simulink model "prova"  (R2023b)
settings: Solver=ode4  StartTime=0.0  StopTime=tf  FixedStep=t_step  RelTol=1e-3
values from neighbouring files (symbols this model uses):
  ARW = ARW*[1 1 1]'    [gyroscope.m]
  bias = bias*[1 1 1]'    [gyroscope.m]
  I = [Ix 0 0; 0 Iy 0; 0 0 Iz]    [gyroscope.m]
  I_inv = inv(I)    [gyroscope.m]
undefined symbols (not defined in the file or in its folder): A_1, A_2, A_3, A_4, A_5, A_6, alpha, DCM_eci_per, e, FS, H0, h_r_0, i, I_RW, I_vector_RW, inc_tot, InitialTrueAnomalyOfEarth, j_b, matrix_RW_config, matrix_RW_config_inv, mu_E, N_1, N_2, N_3, N_4, N_5, N_6, n_e, p, q0, r_1, r_2, r_3, r_4, r_5, r_6, R_E, rho_d1, rho_d2, rho_d3, rho_d4, rho_d5, rho_d6, rho_s1, rho_s2, rho_s3, rho_s4, rho_s5, rho_s6, t_step, th0, ts_sensor, w0, w0_RW, w_E, wMax_RW
libraries: matrix_library x28, simulink x4, dspindex x3, vrlib x2, aerolibutil x1
(part 2 of 2)

== system prova/TRIAD: Attitude determination algebric Method with 2 sensor/Normalize Vector4 ==
  Vector : Inport
  Divide : Product  Inputs=*/
  Normalize Vector : Subsystem  AncestorBlock=LibrarySAD5/Normalize Vector1
  Versor : Outport
  wires:
  Vector/1 -> Normalize Vector/1(Vector), Divide/1
  Divide/1 -> Versor/1
  Normalize Vector/1(Norm) -> Divide/2

== system prova/TRIAD: Attitude determination algebric Method with 2 sensor/Subsystem ==
  note: S1 = 𝑝;
      | 𝑠2 = (𝑝 ∧ 𝑞)/(|𝑝 ∧ 𝑞|);
      | 𝑠3 = 𝑝 ∧ 𝑠2
  versor p (body frame) : Inport
  versor q (body frame) : Inport  Port=2
  Cross Product : matrix_library/Cross Product
  Cross Product1 : matrix_library/Cross Product
  Matrix Concatenate : Concatenate  NumInputs=3  Mode=Multidimensional array  ConcatenateDimension=2
  Normalize Vector3 : Subsystem
  "Matrix S Measurements " : Outport
  wires:
  versor q (body frame)/1 -> Cross Product/2
  Normalize Vector3/1(Versor) -> Matrix Concatenate/2, Cross Product1/2  "s2"
  versor p (body frame)/1 -> Cross Product1/1, Matrix Concatenate/1, Cross Product/1  "s1"
  Cross Product/1 -> Normalize Vector3/1(Vector)
  Cross Product1/1 -> Matrix Concatenate/3  "s3"
  Matrix Concatenate/1 -> "Matrix S Measurements "/1  "Matrix of measure in body frame"

== system prova/TRIAD: Attitude determination algebric Method with 2 sensor/Subsystem1 ==
  versor a (body frame) : Inport
  versor b (body frame) : Inport  Port=2
  Cross Product : matrix_library/Cross Product
  Cross Product1 : matrix_library/Cross Product
  Matrix Concatenate : Concatenate  NumInputs=3  Mode=Multidimensional array  ConcatenateDimension=2
  Normalize Vector3 : Subsystem
  "Matrix V certain model " : Outport
  wires:
  versor b (body frame)/1 -> Cross Product/2
  Normalize Vector3/1(Versor) -> Matrix Concatenate/2, Cross Product1/2  "s2"
  versor a (body frame)/1 -> Cross Product1/1, Matrix Concatenate/1, Cross Product/1  "s1"
  Cross Product/1 -> Normalize Vector3/1(Vector)
  Cross Product1/1 -> Matrix Concatenate/3  "s3"
  Matrix Concatenate/1 -> "Matrix V certain model "/1  "Matrix of measure in body frame"

== system prova/two-body Keplerian dynamics ECI/Integretion of true anomaly ==
  th0 : Inport
  (1-e^2)^(3/2) : Subsystem
  Constant : Constant
  Cos : Trigonometry  Operator=cos
  Divide : Product  Inputs=*/
  Gain : Gain  Gain=e
  Gain1 : Gain  Gain=n_e
  Integrator : Integrator  InitialConditionSource=external
  Product : Product
  Sum : Sum  Inputs=|++
  th : Outport
  wires:
  Sum/1 -> Product/1, Product/2
  Integrator/1 -> th/1, Cos/1  "theta"
  Divide/1 -> Integrator/1
  Constant/1 -> Sum/1
  Product/1 -> Gain1/1
  Cos/1 -> Gain/1
  Gain/1 -> Sum/2
  (1-e^2)^(3/2)/1(Out1) -> Divide/2
  th0/1 -> Integrator/2
  Gain1/1 -> Divide/1

== system prova/two-body Keplerian dynamics ECI/r_perifocal ==
  th : Inport
  Calculation of norm r : Subsystem
  Constant : Constant  Value=0
  Cos : Trigonometry  Operator=cos
  Mux : Mux  Inputs=3
  Product : Product
  Sin : Trigonometry
  r_per : Outport
  wires:
  Constant/1 -> Mux/3
  Cos/1 -> Mux/1
  th/1 -> Calculation of norm r/1(th), Cos/1, Sin/1
  Sin/1 -> Mux/2
  Mux/1 -> Product/1  "r_n"
  Calculation of norm r/1(Norm(r)) -> Product/2
  Product/1 -> r_per/1  "r_n"

== system prova/Calculation of disturbance torque/M of gravity gradient1/Norm of vector ==
  Vector : Inport
  Dot Product : DotProduct  OutDataTypeStr=Inherit: Inherit via internal rule
  Sqrt : Sqrt
  Norm : Outport
  wires:
  Sqrt/1 -> Norm/1
  Vector/1 -> Dot Product/1, Dot Product/2
  Dot Product/1 -> Sqrt/1

== system prova/Calculation of disturbance torque/Solar pressure on 6 faces/Norm of vector ==
  Vector : Inport
  Dot Product : DotProduct  OutDataTypeStr=Inherit: Inherit via internal rule
  Sqrt : Sqrt
  Norm : Outport
  wires:
  Sqrt/1 -> Norm/1
  Vector/1 -> Dot Product/1, Dot Product/2
  Dot Product/1 -> Sqrt/1

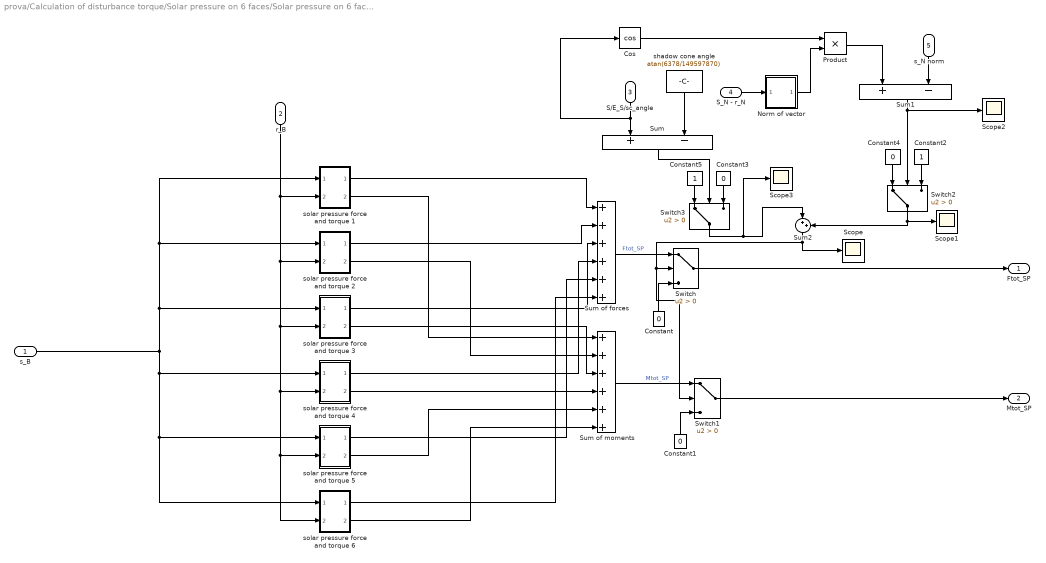
== system prova/Calculation of disturbance torque/Solar pressure on 6 faces/Solar pressure on 6 faces1 ==
  s_B : Inport
  r_B : Inport  Port=2
  S/E_S/sc_angle : Inport  Port=3
  S_N - r_N : Inport  Port=4
  s_N norm : Inport  Port=5
  Constant{,1,3..4} (4 alike) : Constant  Value=0
  Constant2 : Constant
  Constant5 : Constant
  Cos : Trigonometry  Operator=cos
  Norm of vector : Subsystem  AncestorBlock=LibrarySAD5/Normalize Vector1
  Product : Product
  Scope{,1..3} (4 alike) : Scope
  Sum : Sum  Inputs=+-
  Sum of forces : Sum  Inputs=++++++
  Sum of moments : Sum  Inputs=++++++
  Sum1 : Sum  Inputs=+-
  Sum2 : Sum  Inputs=|++
  Switch{,1..3} (4 alike) : Switch  Criteria=u2 > Threshold  SaturateOnIntegerOverflow=off  InputSameDT=off
  shadow cone angle : Constant  Value=atan(6378/149597870)
  solar pressure force and torque 1 : Subsystem
  solar pressure force and torque 2 : Subsystem
  solar pressure force and torque 3 : Subsystem
  solar pressure force and torque 4 : Subsystem
  solar pressure force and torque 5 : Subsystem
  solar pressure force and torque 6 : Subsystem
  Ftot_SP : Outport
  Mtot_SP : Outport  Port=2
  wires:
  s_B/1 -> solar pressure force and torque 1/1(s_B), solar pressure force and torque 2/1(s_B), solar pressure force and torque 3/1(s_B), solar pressure force and torque 4/1(s_B), solar pressure force and torque 6/1(s_B), solar pressure force and torque 5/1(s_B)
  solar pressure force and torque 1/1(F_1) -> Sum of forces/1
  solar pressure force and torque 1/2(M_1) -> Sum of moments/1
  solar pressure force and torque 2/1(F_2) -> Sum of forces/2
  r_B/1 -> solar pressure force and torque 6/2(r_N), solar pressure force and torque 5/2(r_N), solar pressure force and torque 4/2(r_N), solar pressure force and torque 3/2(r_N), solar pressure force and torque 2/2(r_N), solar pressure force and torque 1/2(r_N)
  solar pressure force and torque 2/2(M_2) -> Sum of moments/2
  solar pressure force and torque 3/1(F_3) -> Sum of forces/3
  solar pressure force and torque 3/2(M_3) -> Sum of moments/3
  solar pressure force and torque 4/1(F_4) -> Sum of forces/4
  solar pressure force and torque 4/2(M_4) -> Sum of moments/4
  solar pressure force and torque 5/1(F_5) -> Sum of forces/5
  solar pressure force and torque 5/2(M_5) -> Sum of moments/5
  solar pressure force and torque 6/1(F_6) -> Sum of forces/6
  solar pressure force and torque 6/2(M_6) -> Sum of moments/6
  Sum of forces/1 -> Switch/1  "Ftot_SP"
  Constant/1 -> Switch/3
  S/E_S/sc_angle/1 -> Cos/1, Sum/1
  shadow cone angle/1 -> Sum/2
  Sum of moments/1 -> Switch1/1  "Mtot_SP"
  Constant1/1 -> Switch1/3
  S_N - r_N/1 -> Norm of vector/1(Vector)
  Constant2/1 -> Switch2/3
  Cos/1 -> Product/1
  Norm of vector/1(Norm) -> Product/2
  Product/1 -> Sum1/1
  s_N norm/1 -> Sum1/2
  Sum/1 -> Switch3/2
  Sum1/1 -> Switch2/2, Scope2/1
  Constant4/1 -> Switch2/1
  Constant5/1 -> Switch3/1
  Constant3/1 -> Switch3/3
  Switch3/1 -> Scope3/1, Sum2/1
  Switch2/1 -> Sum2/2, Scope1/1
  Sum2/1 -> Scope/1, Switch1/2, Switch/2
  Switch/1 -> Ftot_SP/1
  Switch1/1 -> Mtot_SP/1

== system prova/Create matrix to statistical method/Normalize Vector1/Normalize Vector ==
  Vector : Inport
  Dot Product : DotProduct  OutDataTypeStr=Inherit: Inherit via internal rule
  Sqrt : Sqrt
  Norm : Outport
  wires:
  Sqrt/1 -> Norm/1
  Vector/1 -> Dot Product/1, Dot Product/2
  Dot Product/1 -> Sqrt/1

== system prova/Create matrix to statistical method/Normalize Vector2/Normalize Vector ==
  Vector : Inport
  Dot Product : DotProduct  OutDataTypeStr=Inherit: Inherit via internal rule
  Sqrt : Sqrt
  Norm : Outport
  wires:
  Sqrt/1 -> Norm/1
  Vector/1 -> Dot Product/1, Dot Product/2
  Dot Product/1 -> Sqrt/1

== system prova/Create matrix to statistical method/Normalize Vector3/Normalize Vector ==
  Vector : Inport
  Dot Product : DotProduct  OutDataTypeStr=Inherit: Inherit via internal rule
  Sqrt : Sqrt
  Norm : Outport
  wires:
  Sqrt/1 -> Norm/1
  Vector/1 -> Dot Product/1, Dot Product/2
  Dot Product/1 -> Sqrt/1

== system prova/Create matrix to statistical method/Normalize Vector4/Normalize Vector ==
  Vector : Inport
  Dot Product : DotProduct  OutDataTypeStr=Inherit: Inherit via internal rule
  Sqrt : Sqrt
  Norm : Outport
  wires:
  Sqrt/1 -> Norm/1
  Vector/1 -> Dot Product/1, Dot Product/2
  Dot Product/1 -> Sqrt/1

== system prova/Dipol Model of Magnetic Field/Calculation of b_n/Norm of Vector ==
  Vector : Inport
  Dot Product : DotProduct  OutDataTypeStr=Inherit: Inherit via internal rule
  Sqrt : Sqrt
  Norm : Outport
  wires:
  Sqrt/1 -> Norm/1
  Vector/1 -> Dot Product/1, Dot Product/2
  Dot Product/1 -> Sqrt/1

== system prova/Dipol Model of Magnetic Field/Calculation of b_n/Norm of Vector H ==
  Vector : Inport
  Dot Product : DotProduct  OutDataTypeStr=Inherit: Inherit via internal rule
  Sqrt : Sqrt
  Norm : Outport
  wires:
  Sqrt/1 -> Norm/1
  Vector/1 -> Dot Product/1, Dot Product/2
  Dot Product/1 -> Sqrt/1

== system prova/Dipol Model of Magnetic Field/Calculation of b_n/Normalize Vector ==
  Vector : Inport
  Divide : Product  Inputs=*/
  Normalize Vector1 : Subsystem  AncestorBlock=LibrarySAD5/Normalize Vector1
  Versor : Outport
  wires:
  Vector/1 -> Normalize Vector1/1(Vector), Divide/1
  Divide/1 -> Versor/1
  Normalize Vector1/1(Norm) -> Divide/2

== system prova/Dipol Model of Magnetic Field/Calculation of b_n/m_versor ==
  Clock : Clock
  Constant : Constant  Value=cos(deg2rad(11.5))
  Cos : Trigonometry  Operator=cos
  Gain : Gain  Gain=deg2rad(w_E)
  Gain1 : Gain  Gain=sin(deg2rad(11.5))
  Gain2 : Gain  Gain=sin(deg2rad(11.5))
  Sin : Trigonometry
  Vector Concatenate : Concatenate  NumInputs=3
  m_versor : Outport
  wires:
  Clock/1 -> Gain/1
  Gain/1 -> Sin/1, Cos/1
  Gain2/1 -> Vector Concatenate/2
  Vector Concatenate/1 -> m_versor/1
  Cos/1 -> Gain1/1
  Constant/1 -> Vector Concatenate/3
  Sin/1 -> Gain2/1
  Gain1/1 -> Vector Concatenate/1

== system prova/Dynamics e Kinematics/Attitude error GG/calculating A_B//L ==
  Theta : Inport
  A_B/N : Inport  Port=2
  Matrix Multiply : Product  Multiplication=Matrix(*)
  Subsystem : Subsystem
  Transpose : Math  Operator=transpose
  A_B/L : Outport
  wires:
  Theta/1 -> Subsystem/1(Theta)
  Transpose/1 -> Matrix Multiply/2
  A_B/N/1 -> Matrix Multiply/1
  Matrix Multiply/1 -> A_B/L/1
  Subsystem/1(" A_L/N") -> Transpose/1

== system prova/Dynamics e Kinematics/DCM composition from quaternions 1/Cross product matrix composition ==
  q_vect : Inport
  Demux : Demux  Outputs=3
  Gain : Gain  Gain=[0 0 0; 0 0 -1; 0 1 0]
  Gain1 : Gain  Gain=[0 0 1; 0 0 0; -1 0 0]
  Gain2 : Gain  Gain=[0 -1 0; 1 0 0; 0 0 0]
  Sum : Sum  Inputs=+++
  q_vect cross : Outport
  wires:
  Gain1/1 -> Sum/2
  Demux/3 -> Gain2/1
  Demux/1 -> Gain/1
  q_vect/1 -> Demux/1
  Gain2/1 -> Sum/3
  Demux/2 -> Gain1/1
  Gain/1 -> Sum/1
  Sum/1 -> q_vect cross/1

== system prova/Dynamics e Kinematics/Kinematics quaternion2/Matrix OMEGA ==
  omega : Inport
  Constant4 : Constant  Value=0
  Demux : Demux  Outputs=3
  Gain : Gain  Gain=-1
  Gain1 : Gain  Gain=-1
  Gain2 : Gain  Gain=-1
  Matrix Concatenate : Concatenate  NumInputs=4  Mode=Multidimensional array  ConcatenateDimension=2
  Vector Concatenate{,2..4} (4 alike) : Concatenate  NumInputs=4
  Matrix Omega : Outport
  wires:
  Demux/2 -> Vector Concatenate4/2, Vector Concatenate/3, Gain1/1  "W_v"
  Gain1/1 -> Vector Concatenate2/4, Vector Concatenate3/1
  Matrix Concatenate/1 -> Matrix Omega/1
  Gain2/1 -> Vector Concatenate3/4, Vector Concatenate/2  "-W_w"
  Vector Concatenate3/1 -> Matrix Concatenate/3
  Demux/3 -> Vector Concatenate2/1, Vector Concatenate4/3, Gain2/1  "W_w"
  Gain/1 -> Vector Concatenate/4, Vector Concatenate2/3  "-W_u"
  Constant4/1 -> Vector Concatenate/1, Vector Concatenate2/2, Vector Concatenate3/3, Vector Concatenate4/4
  Demux/1 -> Vector Concatenate3/2, Vector Concatenate4/1, Gain/1  "W_u"
  Vector Concatenate4/1 -> Matrix Concatenate/4
  Vector Concatenate2/1 -> Matrix Concatenate/2
  Vector Concatenate/1 -> Matrix Concatenate/1
  omega/1 -> Demux/1

== system prova/Dynamics e Kinematics/Kinematics quaternion2/Normalize Vector2 ==
  Vector : Inport
  Dot Product : DotProduct  OutDataTypeStr=Inherit: Inherit via internal rule
  Sqrt : Sqrt
  Norm : Outport
  wires:
  Sqrt/1 -> Norm/1
  Vector/1 -> Dot Product/1, Dot Product/2
  Dot Product/1 -> Sqrt/1

== system prova/Subsystem/DCM to quaternion/Normalize Vector1 ==
  Vector : Inport
  Divide : Product  Inputs=*/
  Norm vector : Subsystem  AncestorBlock=LibrarySAD5/Normalize Vector1
  Versor : Outport
  wires:
  Vector/1 -> Norm vector/1(Vector), Divide/1
  Divide/1 -> Versor/1
  Norm vector/1(Norm) -> Divide/2

== system prova/Subsystem/Normalize Vector1/Norm vector ==
  Vector : Inport
  Dot Product : DotProduct  OutDataTypeStr=Inherit: Inherit via internal rule
  Sqrt : Sqrt
  Norm : Outport
  wires:
  Sqrt/1 -> Norm/1
  Vector/1 -> Dot Product/1, Dot Product/2
  Dot Product/1 -> Sqrt/1

== system prova/Subsystem/Normalize Vector2/Norm vector ==
  Vector : Inport
  Dot Product : DotProduct  OutDataTypeStr=Inherit: Inherit via internal rule
  Sqrt : Sqrt
  Norm : Outport
  wires:
  Sqrt/1 -> Norm/1
  Vector/1 -> Dot Product/1, Dot Product/2
  Dot Product/1 -> Sqrt/1

== system prova/Subsystem/Normalize Vector3/Norm vector ==
  Vector : Inport
  Dot Product : DotProduct  OutDataTypeStr=Inherit: Inherit via internal rule
  Sqrt : Sqrt
  Norm : Outport
  wires:
  Sqrt/1 -> Norm/1
  Vector/1 -> Dot Product/1, Dot Product/2
  Dot Product/1 -> Sqrt/1

== system prova/Subsystem/Normalize Vector4/Norm vector ==
  Vector : Inport
  Dot Product : DotProduct  OutDataTypeStr=Inherit: Inherit via internal rule
  Sqrt : Sqrt
  Norm : Outport
  wires:
  Sqrt/1 -> Norm/1
  Vector/1 -> Dot Product/1, Dot Product/2
  Dot Product/1 -> Sqrt/1

== system prova/Subsystem1/Normalize Vector1/Norm vector ==
  Vector : Inport
  Dot Product : DotProduct  OutDataTypeStr=Inherit: Inherit via internal rule
  Sqrt : Sqrt
  Norm : Outport
  wires:
  Sqrt/1 -> Norm/1
  Vector/1 -> Dot Product/1, Dot Product/2
  Dot Product/1 -> Sqrt/1

== system prova/Sun sensor (Da fare sistmando vettore e eclissi)/Normalize Vector1/Normalize Vector ==
  Vector : Inport
  Dot Product : DotProduct  OutDataTypeStr=Inherit: Inherit via internal rule
  Sqrt : Sqrt
  Norm : Outport
  wires:
  Sqrt/1 -> Norm/1
  Vector/1 -> Dot Product/1, Dot Product/2
  Dot Product/1 -> Sqrt/1

== system prova/TRIAD: Attitude determination algebric Method with 2 sensor/Normalize Vector1/Normalize Vector ==
  Vector : Inport
  Dot Product : DotProduct  OutDataTypeStr=Inherit: Inherit via internal rule
  Sqrt : Sqrt
  Norm : Outport
  wires:
  Sqrt/1 -> Norm/1
  Vector/1 -> Dot Product/1, Dot Product/2
  Dot Product/1 -> Sqrt/1

== system prova/TRIAD: Attitude determination algebric Method with 2 sensor/Normalize Vector2/Norm vector ==
  Vector : Inport
  Dot Product : DotProduct  OutDataTypeStr=Inherit: Inherit via internal rule
  Sqrt : Sqrt
  Norm : Outport
  wires:
  Sqrt/1 -> Norm/1
  Vector/1 -> Dot Product/1, Dot Product/2
  Dot Product/1 -> Sqrt/1

== system prova/TRIAD: Attitude determination algebric Method with 2 sensor/Normalize Vector3/Normalize Vector ==
  Vector : Inport
  Dot Product : DotProduct  OutDataTypeStr=Inherit: Inherit via internal rule
  Sqrt : Sqrt
  Norm : Outport
  wires:
  Sqrt/1 -> Norm/1
  Vector/1 -> Dot Product/1, Dot Product/2
  Dot Product/1 -> Sqrt/1

== system prova/TRIAD: Attitude determination algebric Method with 2 sensor/Normalize Vector4/Normalize Vector ==
  Vector : Inport
  Dot Product : DotProduct  OutDataTypeStr=Inherit: Inherit via internal rule
  Sqrt : Sqrt
  Norm : Outport
  wires:
  Sqrt/1 -> Norm/1
  Vector/1 -> Dot Product/1, Dot Product/2
  Dot Product/1 -> Sqrt/1

== system prova/TRIAD: Attitude determination algebric Method with 2 sensor/Subsystem/Normalize Vector3 ==
  Vector : Inport
  Divide : Product  Inputs=*/
  Normalize Vector : Subsystem  AncestorBlock=LibrarySAD5/Normalize Vector1
  Versor : Outport
  wires:
  Vector/1 -> Normalize Vector/1(Vector), Divide/1
  Divide/1 -> Versor/1
  Normalize Vector/1(Norm) -> Divide/2

== system prova/TRIAD: Attitude determination algebric Method with 2 sensor/Subsystem1/Normalize Vector3 ==
  Vector : Inport
  Divide : Product  Inputs=*/
  Normalize Vector : Subsystem  AncestorBlock=LibrarySAD5/Normalize Vector1
  Versor : Outport
  wires:
  Vector/1 -> Normalize Vector/1(Vector), Divide/1
  Divide/1 -> Versor/1
  Normalize Vector/1(Norm) -> Divide/2

== system prova/two-body Keplerian dynamics ECI/Integretion of true anomaly/(1-e^2)^(3//2) ==
  Constant1 : Constant
  Constant2 : Constant  Value=e
  Constant3 : Constant  Value=3/2
  Power : Math  Operator=pow
  Product1 : Product
  Subtract : Sum  Inputs=+-
  Out1 : Outport
  wires:
  Constant3/1 -> Power/2
  Constant2/1 -> Product1/2, Product1/1
  Subtract/1 -> Power/1
  Constant1/1 -> Subtract/1
  Product1/1 -> Subtract/2
  Power/1 -> Out1/1

== system prova/two-body Keplerian dynamics ECI/r_perifocal/Calculation of norm r ==
  th : Inport
  Constant : Constant  Value=p
  Constant2 : Constant
  Cos : Trigonometry  Operator=cos
  Divide : Product  Inputs=*/
  Gain1 : Gain  Gain=e
  Sum : Sum  Inputs=|++
  Norm(r) : Outport
  wires:
  Constant/1 -> Divide/1
  Gain1/1 -> Sum/2
  Constant2/1 -> Sum/1
  Cos/1 -> Gain1/1
  Sum/1 -> Divide/2
  th/1 -> Cos/1
  Divide/1 -> Norm(r)/1

== system prova/Calculation of disturbance torque/Solar pressure on 6 faces/Solar pressure on 6 faces1/Norm of vector ==
  Vector : Inport
  Dot Product : DotProduct  OutDataTypeStr=Inherit: Inherit via internal rule
  Sqrt : Sqrt
  Norm : Outport
  wires:
  Sqrt/1 -> Norm/1
  Vector/1 -> Dot Product/1, Dot Product/2
  Dot Product/1 -> Sqrt/1

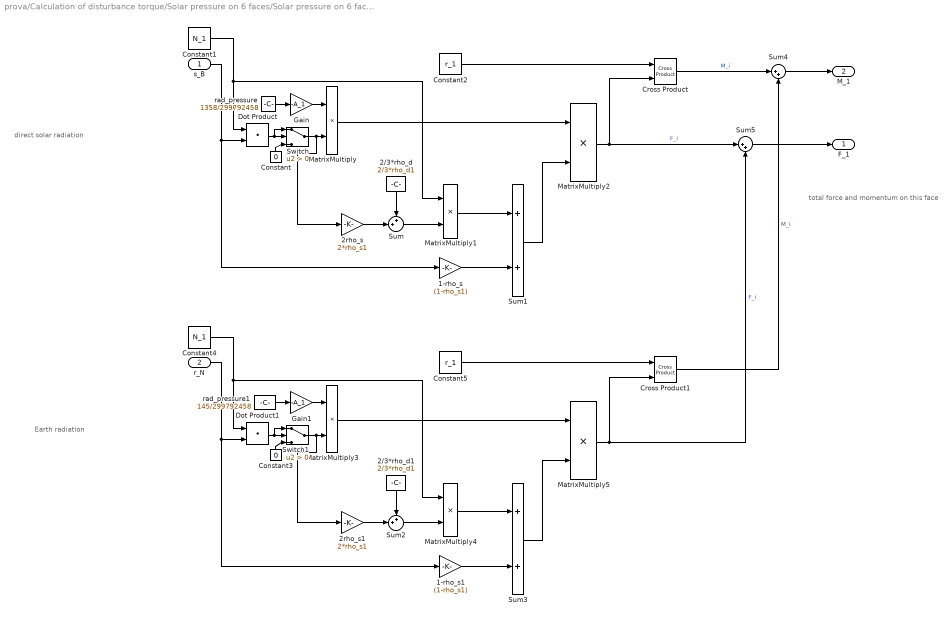
== system prova/Calculation of disturbance torque/Solar pressure on 6 faces/Solar pressure on 6 faces1/solar pressure force and torque 1 ==
  note: total force and
      | momentum on this face
  note: direct solar radiation
  note: Earth radiation
  s_B : Inport
  r_N : Inport  Port=2
  1-rho_s : Gain  Gain=(1-rho_s1)
  1-rho_s1 : Gain  Gain=(1-rho_s1)
  2/3*rho_d : Constant  Value=2/3*rho_d1
  2/3*rho_d1 : Constant  Value=2/3*rho_d1
  2rho_s : Gain  Gain=2*rho_s1
  2rho_s1 : Gain  Gain=2*rho_s1
  Constant : Constant  Value=0
  Constant1 : Constant  Value=N_1
  Constant2 : Constant  Value=r_1
  Constant3 : Constant  Value=0
  Constant4 : Constant  Value=N_1
  Constant5 : Constant  Value=r_1
  Cross Product : matrix_library/Cross Product
  Cross Product1 : matrix_library/Cross Product
  Dot Product : DotProduct  OutDataTypeStr=Inherit: Inherit via internal rule
  Dot Product1 : DotProduct  OutDataTypeStr=Inherit: Inherit via internal rule
  Gain : Gain  Gain=-A_1
  Gain1 : Gain  Gain=-A_1
  MatrixMultiply{,1..5} (6 alike) : Product
  Sum : Sum  Inputs=++|
  Sum1 : Sum
  Sum2 : Sum  Inputs=++|
  Sum3 : Sum
  Sum4 : Sum  Inputs=|++
  Sum5 : Sum  Inputs=|++
  Switch : Switch  Criteria=u2 > Threshold  SaturateOnIntegerOverflow=off  InputSameDT=off
  Switch1 : Switch  Criteria=u2 > Threshold  SaturateOnIntegerOverflow=off  InputSameDT=off
  rad_pressure : Constant  Value=1358/299792458
  rad_pressure1 : Constant  Value=145/299792458
  F_1 : Outport
  M_1 : Outport  Port=2
  wires:
  MatrixMultiply2/1 -> Sum5/1, Cross Product/2  "F_i"
  MatrixMultiply/1 -> MatrixMultiply2/1
  Sum1/1 -> MatrixMultiply2/2
  s_B/1 -> 1-rho_s/1, Dot Product/2
  1-rho_s/1 -> Sum1/2
  rad_pressure/1 -> Gain/1
  MatrixMultiply1/1 -> Sum1/1
  Constant1/1 -> MatrixMultiply1/1, Dot Product/1
  Gain/1 -> MatrixMultiply/1
  Constant2/1 -> Cross Product/1
  Dot Product/1 -> Switch/1, Switch/2
  Constant/1 -> Switch/3
  Switch/1 -> 2rho_s/1, MatrixMultiply/2
  2rho_s/1 -> Sum/2
  2/3*rho_d/1 -> Sum/1
  Sum/1 -> MatrixMultiply1/2
  Sum3/1 -> MatrixMultiply5/2
  r_N/1 -> 1-rho_s1/1, Dot Product1/2
  1-rho_s1/1 -> Sum3/2
  2rho_s1/1 -> Sum2/2
  Switch1/1 -> 2rho_s1/1, MatrixMultiply3/2
  MatrixMultiply4/1 -> Sum3/1
  Constant5/1 -> Cross Product1/1
  MatrixMultiply3/1 -> MatrixMultiply5/1
  rad_pressure1/1 -> Gain1/1
  Constant3/1 -> Switch1/3
  Constant4/1 -> MatrixMultiply4/1, Dot Product1/1
  MatrixMultiply5/1 -> Sum5/2, Cross Product1/2  "F_i"
  Dot Product1/1 -> Switch1/1, Switch1/2
  Cross Product1/1 -> Sum4/2  "M_i"
  Sum2/1 -> MatrixMultiply4/2
  Gain1/1 -> MatrixMultiply3/1
  2/3*rho_d1/1 -> Sum2/1
  Sum4/1 -> M_1/1
  Cross Product/1 -> Sum4/1  "M_i"
  Sum5/1 -> F_1/1

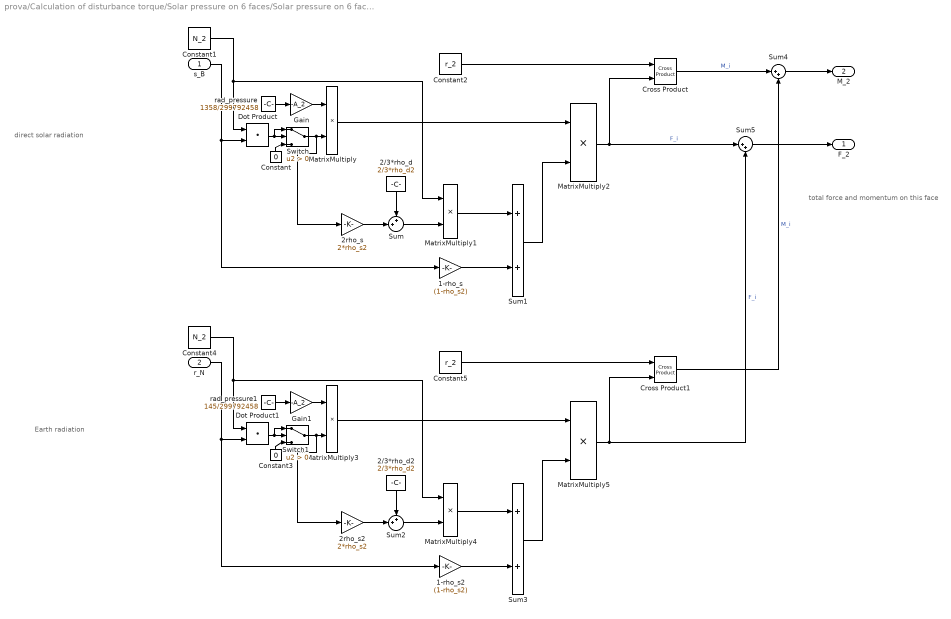
== system prova/Calculation of disturbance torque/Solar pressure on 6 faces/Solar pressure on 6 faces1/solar pressure force and torque 2 ==
  note: total force and
      | momentum on this face
  note: direct solar radiation
  note: Earth radiation
  s_B : Inport
  r_N : Inport  Port=2
  1-rho_s : Gain  Gain=(1-rho_s2)
  1-rho_s2 : Gain  Gain=(1-rho_s2)
  2/3*rho_d : Constant  Value=2/3*rho_d2
  2/3*rho_d2 : Constant  Value=2/3*rho_d2
  2rho_s : Gain  Gain=2*rho_s2
  2rho_s2 : Gain  Gain=2*rho_s2
  Constant : Constant  Value=0
  Constant1 : Constant  Value=N_2
  Constant2 : Constant  Value=r_2
  Constant3 : Constant  Value=0
  Constant4 : Constant  Value=N_2
  Constant5 : Constant  Value=r_2
  Cross Product : matrix_library/Cross Product
  Cross Product1 : matrix_library/Cross Product
  Dot Product : DotProduct  OutDataTypeStr=Inherit: Inherit via internal rule
  Dot Product1 : DotProduct  OutDataTypeStr=Inherit: Inherit via internal rule
  Gain : Gain  Gain=-A_2
  Gain1 : Gain  Gain=-A_2
  MatrixMultiply{,1..5} (6 alike) : Product
  Sum : Sum  Inputs=++|
  Sum1 : Sum
  Sum2 : Sum  Inputs=++|
  Sum3 : Sum
  Sum4 : Sum  Inputs=|++
  Sum5 : Sum  Inputs=|++
  Switch : Switch  Criteria=u2 > Threshold  SaturateOnIntegerOverflow=off  InputSameDT=off
  Switch1 : Switch  Criteria=u2 > Threshold  SaturateOnIntegerOverflow=off  InputSameDT=off
  rad_pressure : Constant  Value=1358/299792458
  rad_pressure1 : Constant  Value=145/299792458
  F_2 : Outport
  M_2 : Outport  Port=2
  wires:
  MatrixMultiply2/1 -> Sum5/1, Cross Product/2  "F_i"
  MatrixMultiply/1 -> MatrixMultiply2/1
  Sum1/1 -> MatrixMultiply2/2
  s_B/1 -> 1-rho_s/1, Dot Product/2
  1-rho_s/1 -> Sum1/2
  rad_pressure/1 -> Gain/1
  MatrixMultiply1/1 -> Sum1/1
  Constant1/1 -> MatrixMultiply1/1, Dot Product/1
  Gain/1 -> MatrixMultiply/1
  Constant2/1 -> Cross Product/1
  Dot Product/1 -> Switch/1, Switch/2
  Constant/1 -> Switch/3
  Switch/1 -> 2rho_s/1, MatrixMultiply/2
  2rho_s/1 -> Sum/2
  2/3*rho_d/1 -> Sum/1
  Sum/1 -> MatrixMultiply1/2
  Sum3/1 -> MatrixMultiply5/2
  r_N/1 -> 1-rho_s2/1, Dot Product1/2
  1-rho_s2/1 -> Sum3/2
  2rho_s2/1 -> Sum2/2
  Switch1/1 -> 2rho_s2/1, MatrixMultiply3/2
  MatrixMultiply4/1 -> Sum3/1
  Constant5/1 -> Cross Product1/1
  MatrixMultiply3/1 -> MatrixMultiply5/1
  rad_pressure1/1 -> Gain1/1
  Constant3/1 -> Switch1/3
  Constant4/1 -> MatrixMultiply4/1, Dot Product1/1
  MatrixMultiply5/1 -> Sum5/2, Cross Product1/2  "F_i"
  Dot Product1/1 -> Switch1/1, Switch1/2
  Cross Product1/1 -> Sum4/2  "M_i"
  Sum2/1 -> MatrixMultiply4/2
  Gain1/1 -> MatrixMultiply3/1
  2/3*rho_d2/1 -> Sum2/1
  Sum4/1 -> M_2/1
  Cross Product/1 -> Sum4/1  "M_i"
  Sum5/1 -> F_2/1

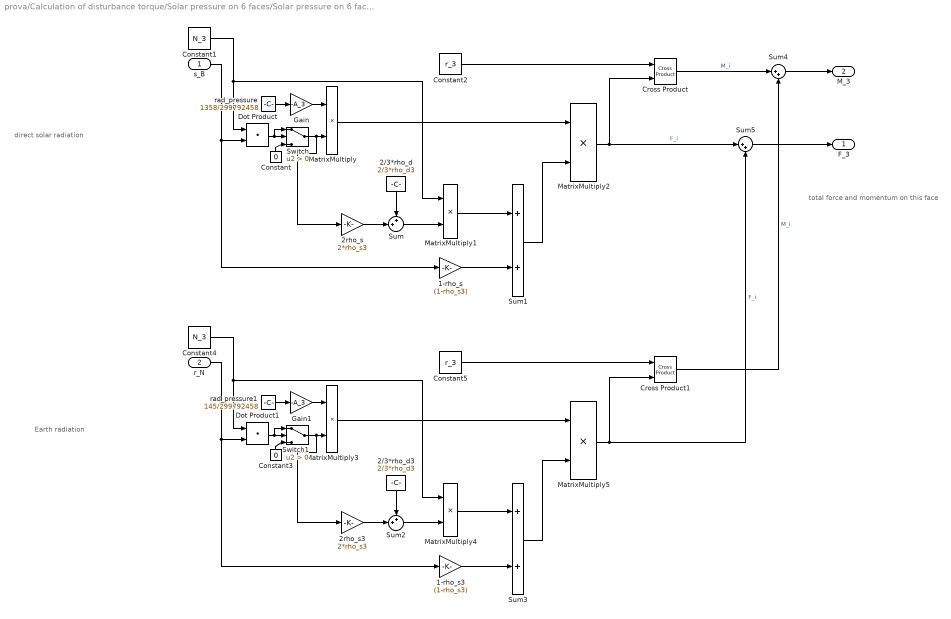
== system prova/Calculation of disturbance torque/Solar pressure on 6 faces/Solar pressure on 6 faces1/solar pressure force and torque 3 ==
  note: total force and
      | momentum on this face
  note: direct solar radiation
  note: Earth radiation
  s_B : Inport
  r_N : Inport  Port=2
  1-rho_s : Gain  Gain=(1-rho_s3)
  1-rho_s3 : Gain  Gain=(1-rho_s3)
  2/3*rho_d : Constant  Value=2/3*rho_d3
  2/3*rho_d3 : Constant  Value=2/3*rho_d3
  2rho_s : Gain  Gain=2*rho_s3
  2rho_s3 : Gain  Gain=2*rho_s3
  Constant : Constant  Value=0
  Constant1 : Constant  Value=N_3
  Constant2 : Constant  Value=r_3
  Constant3 : Constant  Value=0
  Constant4 : Constant  Value=N_3
  Constant5 : Constant  Value=r_3
  Cross Product : matrix_library/Cross Product
  Cross Product1 : matrix_library/Cross Product
  Dot Product : DotProduct  OutDataTypeStr=Inherit: Inherit via internal rule
  Dot Product1 : DotProduct  OutDataTypeStr=Inherit: Inherit via internal rule
  Gain : Gain  Gain=-A_3
  Gain1 : Gain  Gain=-A_3
  MatrixMultiply{,1..5} (6 alike) : Product
  Sum : Sum  Inputs=++|
  Sum1 : Sum
  Sum2 : Sum  Inputs=++|
  Sum3 : Sum
  Sum4 : Sum  Inputs=|++
  Sum5 : Sum  Inputs=|++
  Switch : Switch  Criteria=u2 > Threshold  SaturateOnIntegerOverflow=off  InputSameDT=off
  Switch1 : Switch  Criteria=u2 > Threshold  SaturateOnIntegerOverflow=off  InputSameDT=off
  rad_pressure : Constant  Value=1358/299792458
  rad_pressure1 : Constant  Value=145/299792458
  F_3 : Outport
  M_3 : Outport  Port=2
  wires:
  MatrixMultiply2/1 -> Sum5/1, Cross Product/2  "F_i"
  MatrixMultiply/1 -> MatrixMultiply2/1
  Sum1/1 -> MatrixMultiply2/2
  s_B/1 -> 1-rho_s/1, Dot Product/2
  1-rho_s/1 -> Sum1/2
  rad_pressure/1 -> Gain/1
  MatrixMultiply1/1 -> Sum1/1
  Constant1/1 -> MatrixMultiply1/1, Dot Product/1
  Gain/1 -> MatrixMultiply/1
  Constant2/1 -> Cross Product/1
  Dot Product/1 -> Switch/1, Switch/2
  Constant/1 -> Switch/3
  Switch/1 -> 2rho_s/1, MatrixMultiply/2
  2rho_s/1 -> Sum/2
  2/3*rho_d/1 -> Sum/1
  Sum/1 -> MatrixMultiply1/2
  Sum3/1 -> MatrixMultiply5/2
  r_N/1 -> 1-rho_s3/1, Dot Product1/2
  1-rho_s3/1 -> Sum3/2
  2rho_s3/1 -> Sum2/2
  Switch1/1 -> 2rho_s3/1, MatrixMultiply3/2
  MatrixMultiply4/1 -> Sum3/1
  Constant5/1 -> Cross Product1/1
  MatrixMultiply3/1 -> MatrixMultiply5/1
  rad_pressure1/1 -> Gain1/1
  Constant3/1 -> Switch1/3
  Constant4/1 -> MatrixMultiply4/1, Dot Product1/1
  MatrixMultiply5/1 -> Sum5/2, Cross Product1/2  "F_i"
  Dot Product1/1 -> Switch1/1, Switch1/2
  Cross Product1/1 -> Sum4/2  "M_i"
  Sum2/1 -> MatrixMultiply4/2
  Gain1/1 -> MatrixMultiply3/1
  2/3*rho_d3/1 -> Sum2/1
  Sum4/1 -> M_3/1
  Cross Product/1 -> Sum4/1  "M_i"
  Sum5/1 -> F_3/1

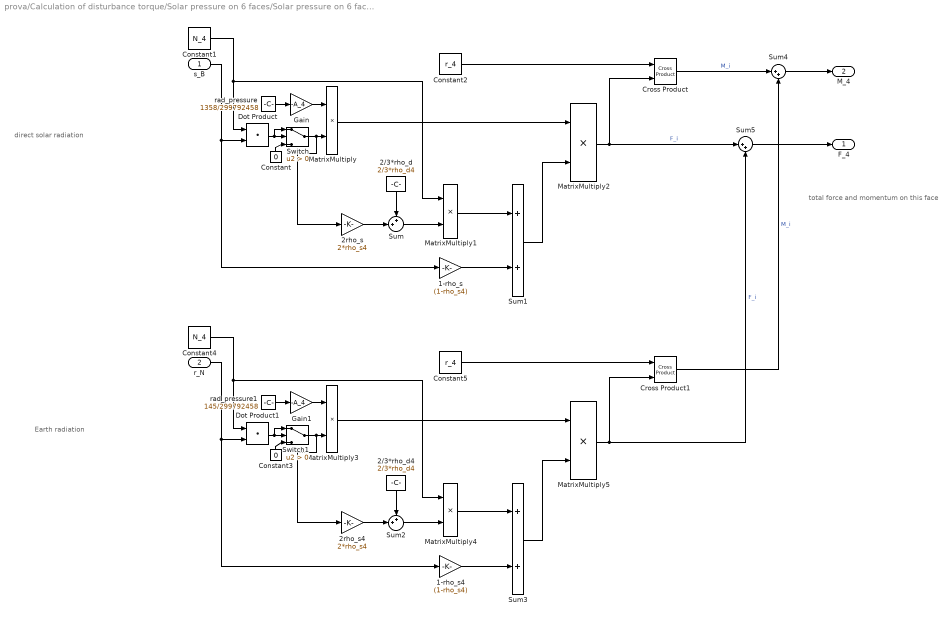
== system prova/Calculation of disturbance torque/Solar pressure on 6 faces/Solar pressure on 6 faces1/solar pressure force and torque 4 ==
  note: total force and
      | momentum on this face
  note: direct solar radiation
  note: Earth radiation
  s_B : Inport
  r_N : Inport  Port=2
  1-rho_s : Gain  Gain=(1-rho_s4)
  1-rho_s4 : Gain  Gain=(1-rho_s4)
  2/3*rho_d : Constant  Value=2/3*rho_d4
  2/3*rho_d4 : Constant  Value=2/3*rho_d4
  2rho_s : Gain  Gain=2*rho_s4
  2rho_s4 : Gain  Gain=2*rho_s4
  Constant : Constant  Value=0
  Constant1 : Constant  Value=N_4
  Constant2 : Constant  Value=r_4
  Constant3 : Constant  Value=0
  Constant4 : Constant  Value=N_4
  Constant5 : Constant  Value=r_4
  Cross Product : matrix_library/Cross Product
  Cross Product1 : matrix_library/Cross Product
  Dot Product : DotProduct  OutDataTypeStr=Inherit: Inherit via internal rule
  Dot Product1 : DotProduct  OutDataTypeStr=Inherit: Inherit via internal rule
  Gain : Gain  Gain=-A_4
  Gain1 : Gain  Gain=-A_4
  MatrixMultiply{,1..5} (6 alike) : Product
  Sum : Sum  Inputs=++|
  Sum1 : Sum
  Sum2 : Sum  Inputs=++|
  Sum3 : Sum
  Sum4 : Sum  Inputs=|++
  Sum5 : Sum  Inputs=|++
  Switch : Switch  Criteria=u2 > Threshold  SaturateOnIntegerOverflow=off  InputSameDT=off
  Switch1 : Switch  Criteria=u2 > Threshold  SaturateOnIntegerOverflow=off  InputSameDT=off
  rad_pressure : Constant  Value=1358/299792458
  rad_pressure1 : Constant  Value=145/299792458
  F_4 : Outport
  M_4 : Outport  Port=2
  wires:
  MatrixMultiply2/1 -> Sum5/1, Cross Product/2  "F_i"
  MatrixMultiply/1 -> MatrixMultiply2/1
  Sum1/1 -> MatrixMultiply2/2
  s_B/1 -> 1-rho_s/1, Dot Product/2
  1-rho_s/1 -> Sum1/2
  rad_pressure/1 -> Gain/1
  MatrixMultiply1/1 -> Sum1/1
  Constant1/1 -> MatrixMultiply1/1, Dot Product/1
  Gain/1 -> MatrixMultiply/1
  Constant2/1 -> Cross Product/1
  Dot Product/1 -> Switch/1, Switch/2
  Constant/1 -> Switch/3
  Switch/1 -> 2rho_s/1, MatrixMultiply/2
  2rho_s/1 -> Sum/2
  2/3*rho_d/1 -> Sum/1
  Sum/1 -> MatrixMultiply1/2
  Sum3/1 -> MatrixMultiply5/2
  r_N/1 -> 1-rho_s4/1, Dot Product1/2
  1-rho_s4/1 -> Sum3/2
  2rho_s4/1 -> Sum2/2
  Switch1/1 -> 2rho_s4/1, MatrixMultiply3/2
  MatrixMultiply4/1 -> Sum3/1
  Constant5/1 -> Cross Product1/1
  MatrixMultiply3/1 -> MatrixMultiply5/1
  rad_pressure1/1 -> Gain1/1
  Constant3/1 -> Switch1/3
  Constant4/1 -> MatrixMultiply4/1, Dot Product1/1
  MatrixMultiply5/1 -> Sum5/2, Cross Product1/2  "F_i"
  Dot Product1/1 -> Switch1/1, Switch1/2
  Cross Product1/1 -> Sum4/2  "M_i"
  Sum2/1 -> MatrixMultiply4/2
  Gain1/1 -> MatrixMultiply3/1
  2/3*rho_d4/1 -> Sum2/1
  Sum4/1 -> M_4/1
  Cross Product/1 -> Sum4/1  "M_i"
  Sum5/1 -> F_4/1

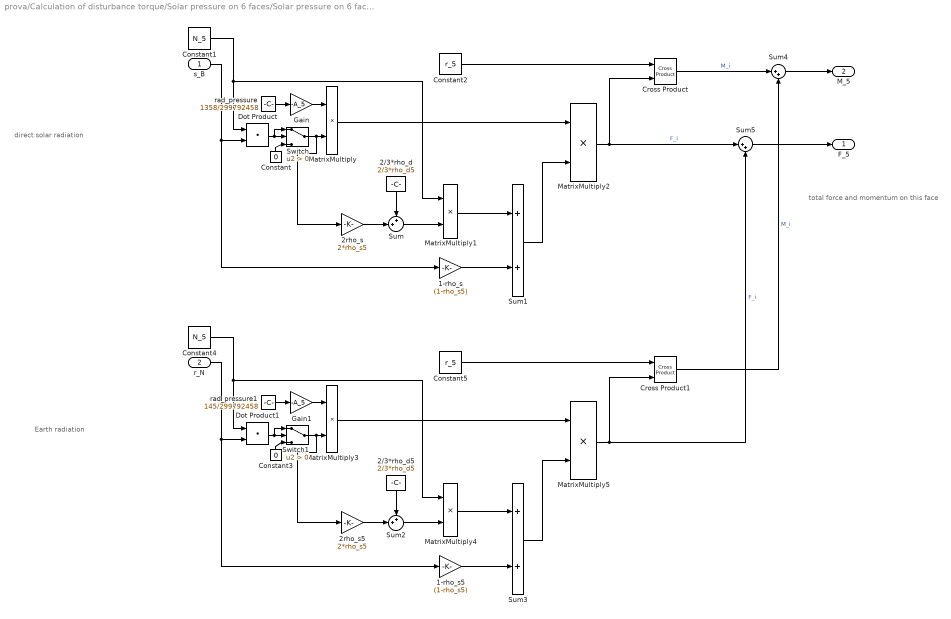
== system prova/Calculation of disturbance torque/Solar pressure on 6 faces/Solar pressure on 6 faces1/solar pressure force and torque 5 ==
  note: total force and
      | momentum on this face
  note: direct solar radiation
  note: Earth radiation
  s_B : Inport
  r_N : Inport  Port=2
  1-rho_s : Gain  Gain=(1-rho_s5)
  1-rho_s5 : Gain  Gain=(1-rho_s5)
  2/3*rho_d : Constant  Value=2/3*rho_d5
  2/3*rho_d5 : Constant  Value=2/3*rho_d5
  2rho_s : Gain  Gain=2*rho_s5
  2rho_s5 : Gain  Gain=2*rho_s5
  Constant : Constant  Value=0
  Constant1 : Constant  Value=N_5
  Constant2 : Constant  Value=r_5
  Constant3 : Constant  Value=0
  Constant4 : Constant  Value=N_5
  Constant5 : Constant  Value=r_5
  Cross Product : matrix_library/Cross Product
  Cross Product1 : matrix_library/Cross Product
  Dot Product : DotProduct  OutDataTypeStr=Inherit: Inherit via internal rule
  Dot Product1 : DotProduct  OutDataTypeStr=Inherit: Inherit via internal rule
  Gain : Gain  Gain=-A_5
  Gain1 : Gain  Gain=-A_5
  MatrixMultiply{,1..5} (6 alike) : Product
  Sum : Sum  Inputs=++|
  Sum1 : Sum
  Sum2 : Sum  Inputs=++|
  Sum3 : Sum
  Sum4 : Sum  Inputs=|++
  Sum5 : Sum  Inputs=|++
  Switch : Switch  Criteria=u2 > Threshold  SaturateOnIntegerOverflow=off  InputSameDT=off
  Switch1 : Switch  Criteria=u2 > Threshold  SaturateOnIntegerOverflow=off  InputSameDT=off
  rad_pressure : Constant  Value=1358/299792458
  rad_pressure1 : Constant  Value=145/299792458
  F_5 : Outport
  M_5 : Outport  Port=2
  wires:
  MatrixMultiply2/1 -> Sum5/1, Cross Product/2  "F_i"
  MatrixMultiply/1 -> MatrixMultiply2/1
  Sum1/1 -> MatrixMultiply2/2
  s_B/1 -> 1-rho_s/1, Dot Product/2
  1-rho_s/1 -> Sum1/2
  rad_pressure/1 -> Gain/1
  MatrixMultiply1/1 -> Sum1/1
  Constant1/1 -> MatrixMultiply1/1, Dot Product/1
  Gain/1 -> MatrixMultiply/1
  Constant2/1 -> Cross Product/1
  Dot Product/1 -> Switch/1, Switch/2
  Constant/1 -> Switch/3
  Switch/1 -> 2rho_s/1, MatrixMultiply/2
  2rho_s/1 -> Sum/2
  2/3*rho_d/1 -> Sum/1
  Sum/1 -> MatrixMultiply1/2
  Sum3/1 -> MatrixMultiply5/2
  r_N/1 -> 1-rho_s5/1, Dot Product1/2
  1-rho_s5/1 -> Sum3/2
  2rho_s5/1 -> Sum2/2
  Switch1/1 -> 2rho_s5/1, MatrixMultiply3/2
  MatrixMultiply4/1 -> Sum3/1
  Constant5/1 -> Cross Product1/1
  MatrixMultiply3/1 -> MatrixMultiply5/1
  rad_pressure1/1 -> Gain1/1
  Constant3/1 -> Switch1/3
  Constant4/1 -> MatrixMultiply4/1, Dot Product1/1
  MatrixMultiply5/1 -> Sum5/2, Cross Product1/2  "F_i"
  Dot Product1/1 -> Switch1/1, Switch1/2
  Cross Product1/1 -> Sum4/2  "M_i"
  Sum2/1 -> MatrixMultiply4/2
  Gain1/1 -> MatrixMultiply3/1
  2/3*rho_d5/1 -> Sum2/1
  Sum4/1 -> M_5/1
  Cross Product/1 -> Sum4/1  "M_i"
  Sum5/1 -> F_5/1

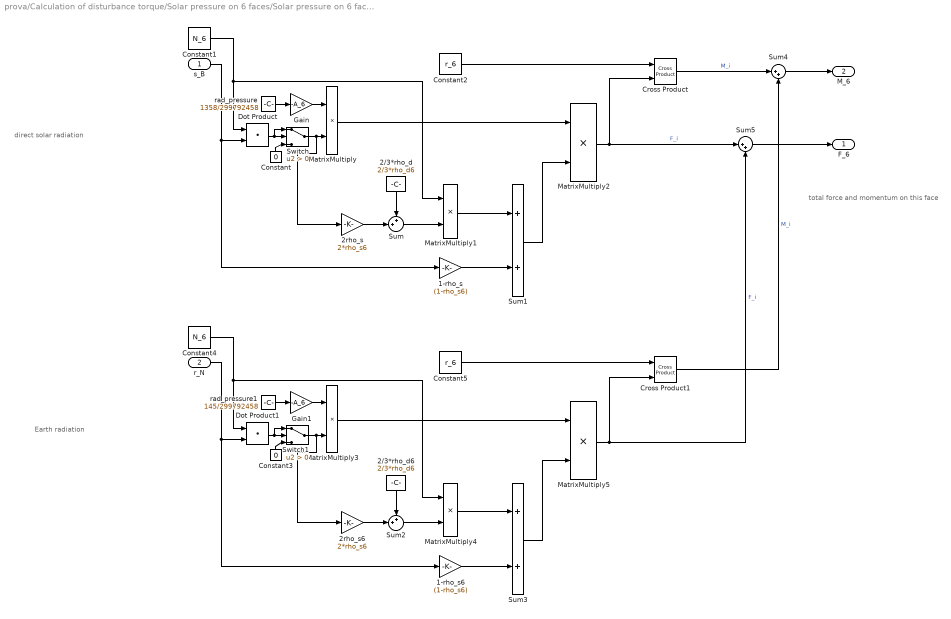
== system prova/Calculation of disturbance torque/Solar pressure on 6 faces/Solar pressure on 6 faces1/solar pressure force and torque 6 ==
  note: total force and
      | momentum on this face
  note: direct solar radiation
  note: Earth radiation
  s_B : Inport
  r_N : Inport  Port=2
  1-rho_s : Gain  Gain=(1-rho_s6)
  1-rho_s6 : Gain  Gain=(1-rho_s6)
  2/3*rho_d : Constant  Value=2/3*rho_d6
  2/3*rho_d6 : Constant  Value=2/3*rho_d6
  2rho_s : Gain  Gain=2*rho_s6
  2rho_s6 : Gain  Gain=2*rho_s6
  Constant : Constant  Value=0
  Constant1 : Constant  Value=N_6
  Constant2 : Constant  Value=r_6
  Constant3 : Constant  Value=0
  Constant4 : Constant  Value=N_6
  Constant5 : Constant  Value=r_6
  Cross Product : matrix_library/Cross Product
  Cross Product1 : matrix_library/Cross Product
  Dot Product : DotProduct  OutDataTypeStr=Inherit: Inherit via internal rule
  Dot Product1 : DotProduct  OutDataTypeStr=Inherit: Inherit via internal rule
  Gain : Gain  Gain=-A_6
  Gain1 : Gain  Gain=-A_6
  MatrixMultiply{,1..5} (6 alike) : Product
  Sum : Sum  Inputs=++|
  Sum1 : Sum
  Sum2 : Sum  Inputs=++|
  Sum3 : Sum
  Sum4 : Sum  Inputs=|++
  Sum5 : Sum  Inputs=|++
  Switch : Switch  Criteria=u2 > Threshold  SaturateOnIntegerOverflow=off  InputSameDT=off
  Switch1 : Switch  Criteria=u2 > Threshold  SaturateOnIntegerOverflow=off  InputSameDT=off
  rad_pressure : Constant  Value=1358/299792458
  rad_pressure1 : Constant  Value=145/299792458
  F_6 : Outport
  M_6 : Outport  Port=2
  wires:
  MatrixMultiply2/1 -> Sum5/1, Cross Product/2  "F_i"
  MatrixMultiply/1 -> MatrixMultiply2/1
  Sum1/1 -> MatrixMultiply2/2
  s_B/1 -> 1-rho_s/1, Dot Product/2
  1-rho_s/1 -> Sum1/2
  rad_pressure/1 -> Gain/1
  MatrixMultiply1/1 -> Sum1/1
  Constant1/1 -> MatrixMultiply1/1, Dot Product/1
  Gain/1 -> MatrixMultiply/1
  Constant2/1 -> Cross Product/1
  Dot Product/1 -> Switch/1, Switch/2
  Constant/1 -> Switch/3
  Switch/1 -> 2rho_s/1, MatrixMultiply/2
  2rho_s/1 -> Sum/2
  2/3*rho_d/1 -> Sum/1
  Sum/1 -> MatrixMultiply1/2
  Sum3/1 -> MatrixMultiply5/2
  r_N/1 -> 1-rho_s6/1, Dot Product1/2
  1-rho_s6/1 -> Sum3/2
  2rho_s6/1 -> Sum2/2
  Switch1/1 -> 2rho_s6/1, MatrixMultiply3/2
  MatrixMultiply4/1 -> Sum3/1
  Constant5/1 -> Cross Product1/1
  MatrixMultiply3/1 -> MatrixMultiply5/1
  rad_pressure1/1 -> Gain1/1
  Constant3/1 -> Switch1/3
  Constant4/1 -> MatrixMultiply4/1, Dot Product1/1
  MatrixMultiply5/1 -> Sum5/2, Cross Product1/2  "F_i"
  Dot Product1/1 -> Switch1/1, Switch1/2
  Cross Product1/1 -> Sum4/2  "M_i"
  Sum2/1 -> MatrixMultiply4/2
  Gain1/1 -> MatrixMultiply3/1
  2/3*rho_d6/1 -> Sum2/1
  Sum4/1 -> M_6/1
  Cross Product/1 -> Sum4/1  "M_i"
  Sum5/1 -> F_6/1

== system prova/Dipol Model of Magnetic Field/Calculation of b_n/Normalize Vector/Normalize Vector1 ==
  Vector : Inport
  Dot Product : DotProduct  OutDataTypeStr=Inherit: Inherit via internal rule
  Sqrt : Sqrt
  Norm : Outport
  wires:
  Sqrt/1 -> Norm/1
  Vector/1 -> Dot Product/1, Dot Product/2
  Dot Product/1 -> Sqrt/1

== system prova/Dynamics e Kinematics/Attitude error GG/calculating A_B//L/Subsystem ==
  Theta : Inport
  Constant : Constant  Value=[1,0,0;0 cos(i) sin(i); 0 -sin(i) cos(i)]
  Constant1 : Constant
  Constant2 : Constant  Value=0
  Cos : Trigonometry  Operator=cos
  Gain : Gain  Gain=-1
  Matrix Concatenate : Concatenate  NumInputs=3  Mode=Multidimensional array  ConcatenateDimension=2
  Matrix Multiply : Product  Multiplication=Matrix(*)
  Sin : Trigonometry
  Vector Concatenate : Concatenate  NumInputs=3
  Vector Concatenate1 : Concatenate  NumInputs=3
  Vector Concatenate2 : Concatenate  NumInputs=3
  " A_L/N" : Outport
  wires:
  Vector Concatenate/1 -> Matrix Concatenate/1
  Vector Concatenate2/1 -> Matrix Concatenate/3
  Matrix Concatenate/1 -> Matrix Multiply/1
  Matrix Multiply/1 -> " A_L/N"/1
  Sin/1 -> Gain/1, Vector Concatenate1/1
  Theta/1 -> Cos/1, Sin/1
  Gain/1 -> Vector Concatenate/2
  Vector Concatenate1/1 -> Matrix Concatenate/2
  Cos/1 -> Vector Concatenate/1, Vector Concatenate1/2
  Constant1/1 -> Vector Concatenate2/3
  Constant/1 -> Matrix Multiply/2
  Constant2/1 -> Vector Concatenate/3, Vector Concatenate1/3, Vector Concatenate2/1, Vector Concatenate2/2

== system prova/Subsystem/DCM to quaternion/Normalize Vector1/Norm vector ==
  Vector : Inport
  Dot Product : DotProduct  OutDataTypeStr=Inherit: Inherit via internal rule
  Sqrt : Sqrt
  Norm : Outport
  wires:
  Sqrt/1 -> Norm/1
  Vector/1 -> Dot Product/1, Dot Product/2
  Dot Product/1 -> Sqrt/1

== system prova/TRIAD: Attitude determination algebric Method with 2 sensor/Subsystem/Normalize Vector3/Normalize Vector ==
  Vector : Inport
  Dot Product : DotProduct  OutDataTypeStr=Inherit: Inherit via internal rule
  Sqrt : Sqrt
  Norm : Outport
  wires:
  Sqrt/1 -> Norm/1
  Vector/1 -> Dot Product/1, Dot Product/2
  Dot Product/1 -> Sqrt/1

== system prova/TRIAD: Attitude determination algebric Method with 2 sensor/Subsystem1/Normalize Vector3/Normalize Vector ==
  Vector : Inport
  Dot Product : DotProduct  OutDataTypeStr=Inherit: Inherit via internal rule
  Sqrt : Sqrt
  Norm : Outport
  wires:
  Sqrt/1 -> Norm/1
  Vector/1 -> Dot Product/1, Dot Product/2
  Dot Product/1 -> Sqrt/1

== matlab function prova/Statistical methods attitude determination (quaternion  Wabha’s problem) /Blocco da convertire in formato simulink. Ho trovato 3 soluzioni differenti al proble ==
  data: K input; q output; S input; Sadj input
function q = fcn(K, S, Sadj)
    
    A = eig(K);
    A = real(A);
    lambda = max(A);
    z = K(1:3, 4);

    %{
    FUNZIONAAA
    %proposta wikipedia
    sigma = 1/2*trace(S);
    %Sadj = det(S)*eye(3)*inv(S);
    k = trace(Sadj);
    delta = det(S);
    alpha = lambda^2 - sigma^2 + k;
    beta = lambda - sigma;
    gamma = (lambda + sigma)*alpha - delta;
    
    x = (alpha*eye(3) + beta*S + S^2)*z;
    
    q =[x; gamma]/sqrt(gamma^2 + norm(x)^2);
    %}
   
    %
    %Proposta libro: FUNZIONAAAAAA -> sceglierei questa: è facile da
    %implementare
    
    z = K(1:3, 4);
    sigma = K(4,4);
    
    mat = (lambda + sigma)*eye(3) - S;
    q = zeros(4,1);
    q(1:3) = (det(mat)*eye(3)*inv(mat)) * z;
    q(4) = det(mat);
    q = q/norm(q);
    %}


    %{
    GIUSTA FUNZIONA, ma restituisce gibbs vector
    z = K(1:3, 4);
    sigma = K(4,4);
    %K = K - eye(4)*lambda;
    
    % linear system
    %Z = zeros(4,1);
    %q = K\Z;
    %q = q/norm(q);
    
    g = (S-(sigma+lambda)*eye(3)) \ (-z);
    
    DCM = [1+g(1)^2-g(2)^2-g(3)^2, 2*(g(1)*g(2)+g(3))    ,  2*(g(1)*g(3)-g(2));
         2*(g(1)*g(2)-g(3))    , 1-g(1)^2+g(2)^2-g(3)^2,  2*(g(2)*g(3)+g(1));
         2*(g(1)*g(3)+g(2))    , 2*(g(2)*g(3)-g(1))    ,  1-g(1)^2-g(2)^2+g(3)^2];
    DCM = DCM./(1+g(1)^2+g(2)^2+g(3)^2);
    %}

    %{
    % soluzione nelle slide, ma la matrice è singolare
    q = (K - lambda*eye(4)) \ zeros(4,1);
    q = q/norm(q);
    %}

end

== matlab function prova/Ouput DCM with gibbs vector (ver slide) ==
  data: alpha input; DCM output; s input; v input
function DCM = fcn(alpha, s, v)

B = zeros(3,3);
K = zeros(4,4);
%
for i = 1:size(s,2)
    B = B + alpha(i)*s(:,i)*v(:,i)';
end

S = B' + B;

z = [B(2,3) - B(3,2), B(3,1) - B(1,3), B(1,2) - B(2,1)]';
sigma = trace(B);
K(1:3, 1:3) = S-eye(3,3)*sigma;
K(1:3,4) = z;
K(4, 1:3) = z';
K(4,4) = sigma;

A = eig(K);
A = real(A);
lambda = max(A);
%K = K - eye(4)*lambda;

% linear system
%Z = zeros(4,1);
%q = K\Z;
%q = q/norm(q);

g = (S-(sigma+lambda)*eye(3)) \ (-z);

DCM = [1+g(1)^2-g(2)^2-g(3)^2, 2*(g(1)*g(2)+g(3))    ,  2*(g(1)*g(3)-g(2));
     2*(g(1)*g(2)-g(3))    , 1-g(1)^2+g(2)^2-g(3)^2,  2*(g(2)*g(3)+g(1));
     2*(g(1)*g(3)+g(2))    , 2*(g(2)*g(3)-g(1))    ,  1-g(1)^2-g(2)^2+g(3)^2];
DCM = DCM./(1+g(1)^2+g(2)^2+g(3)^2);

end
